simulink model "RefModel_Task"  (R2020a)
settings: Solver=ode1  StartTime=0.0  StopTime=10.0  FixedStep=Ts_Task.Ts_base  RelTol=1e-3
undefined symbols (not defined in the file or in its folder): groundspeedCmd, heightCmd, rollCmd
(part 1 of 5)
settings Model: PauseTimes=794.1  OrderedModelArguments=off  Creator=sl  LastModifiedBy=Administrator
settings DataIOCC: SaveOutput=off  SaveTime=off
settings OptimizationCC: DefaultParameterBehavior=Inlined  EnhancedBackFolding=on  PassReuseOutputArgsAs=Individual arguments  ZeroExternalMemoryAtStartup=off  ZeroInternalMemoryAtStartup=off  OptimizeBlockOrder=speed  DifferentSizesBufferReuse=on  OptimizationCustomize=off  EfficientTunableParamExpr=on
settings DebuggingCC: InheritedTsInSrcMsg=none  ParameterPrecisionLossMsg=none  ParameterTunabilityLossMsg=error  UnconnectedInputMsg=none  UnconnectedOutputMsg=none  UnconnectedLineMsg=none  SFUnusedDataAndEventsDiag=none
settings HardwareCC: ProdBitPerPointer=32  ProdBitPerSizeT=32  ProdBitPerPtrDiffT=32  ProdLargestAtomicInteger=Long  ProdLargestAtomicFloat=Double  ProdWordSize=32  ProdHWDeviceType=ARM Compatible->ARM Cortex
settings ModelReferenceCC: ModelReferenceNumInstancesAllowed=Single  PropagateVarSize=During execution
settings SFSimCC: MATLABDynamicMemAlloc=off
settings RTWCC: SystemTargetFile=ert.tlc  TemplateMakefile=ert_default_tmf  GenerateReport=on  IncludeHyperlinkInReport=on  LaunchReport=on  GenerateTraceInfo=on  GenerateTraceReport=on  GenerateTraceReportSl=on  GenerateTraceReportSf=on  GenerateTraceReportEml=on
settings CodeAppCC: ForceParamTrailComments=on  IgnoreCustomStorageClasses=off  MaxIdLength=48  OperatorAnnotations=on  SimulinkDataObjDesc=on  SFDataObjDesc=on  MATLABFcnDesc=on  InsertBlockDesc=on  StateflowObjectComments=on  MATLABSourceComments=on
settings ERTTargetCC: TargetLangStandard=C99 (ISO)  GenerateSampleERTMain=on  CombineOutputUpdateFcns=off  LogVarNameModifier=none  SupportVariableSizeSignals=on  InlinedParameterPlacement=NonHierarchical  ERTCustomFileTemplate=example_file_process.tlc

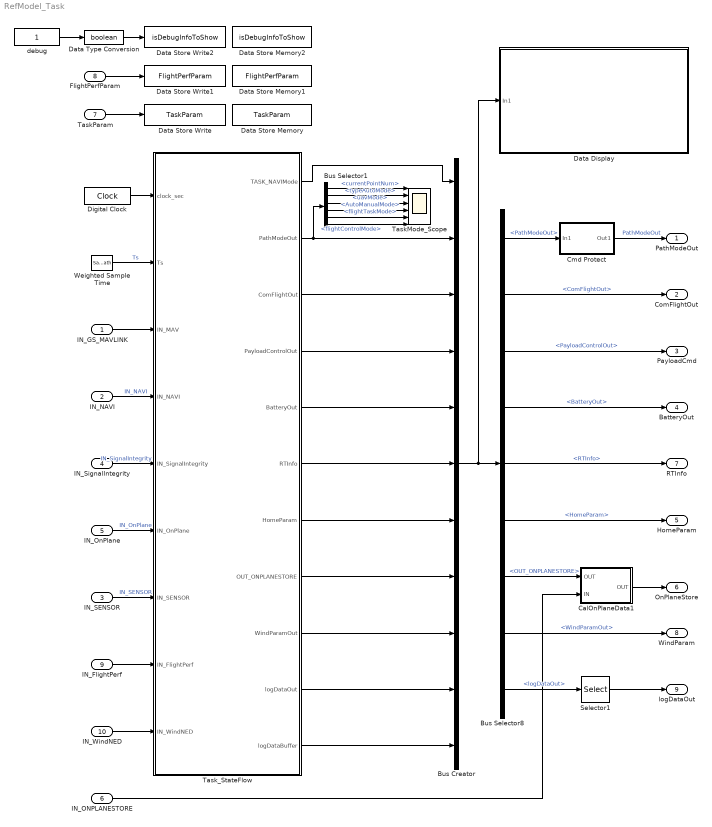
== system RefModel_Task ==
  IN_GS_MAVLINK : Inport  OutDataTypeStr=Bus: BUS_MAVLINK_TO_FIRM  BusOutputAsStruct=on
  IN_NAVI : Inport  Port=2  OutDataTypeStr=Bus: BUS_NAVI_TO_FIRM  BusOutputAsStruct=on
  IN_SENSOR : Inport  Port=3  OutDataTypeStr=Bus: BUS_SENSOR  BusOutputAsStruct=on
  IN_SignalIntegrity : Inport  Port=4  OutDataTypeStr=Bus: BUS_NAVI_SensorSignalIntegrity  BusOutputAsStruct=on
  IN_OnPlane : Inport  Port=5  OutDataTypeStr=Bus: BUS_ONPLANE_FEEDBACK  BusOutputAsStruct=on
  IN_ONPLANESTORE : Inport  Port=6  OutDataTypeStr=Bus: BUS_ONPLANE_STORE  BusOutputAsStruct=on
  TaskParam : Inport  Port=7  OutDataTypeStr=Bus: BUS_TASK_PATH_AlgoParam  BusOutputAsStruct=on
  FlightPerfParam : Inport  Port=8  OutDataTypeStr=Bus: BUS_FLIGHTPERF_PARAM  BusOutputAsStruct=on
  IN_FlightPerf : Inport  Port=9  OutDataTypeStr=Bus: BUS_FLIGHTPERF_OUT  BusOutputAsStruct=on
  IN_WindNED : Inport  Port=10  OutDataTypeStr=Bus: BUS_NAVI_GlobalWindEst
  Bus Creator : BusCreator  Inputs=11
  Bus Selector1 : BusSelector  OutputSignals=currentPointNum,typeAutoMode,uavMode,AutoManualMode,flightTaskMode,flightControlMode
  Bus Selector8 : BusSelector  OutputSignals=PathModeOut,ComFlightOut,PayloadControlOut,BatteryOut,RTInfo,HomeParam,OUT_ONPLANESTORE,WindParamOut,logDataOut
  CalOnPlaneData1 : MATLAB Function  TreatAsAtomicUnit=on
  Cmd Protect : Subsystem
  Data Display : Subsystem
      mask Display: image('$imagefile'); % Use "Edit Image" on toolstrip to change.
  Data Store Memory : DataStoreMemory  DataStoreName=TaskParam  ReadBeforeWriteMsg=warning  WriteAfterWriteMsg=warning  WriteAfterReadMsg=warning  ShowAdditionalParam=off  OutDataTypeStr=Bus: BUS_TASK_PATH_AlgoParam  Dimensions=1
  Data Store Memory1 : DataStoreMemory  DataStoreName=FlightPerfParam  ReadBeforeWriteMsg=warning  WriteAfterWriteMsg=warning  WriteAfterReadMsg=warning  ShowAdditionalParam=off  OutDataTypeStr=Bus: BUS_FLIGHTPERF_PARAM  Dimensions=1
  Data Store Memory2 : DataStoreMemory  DataStoreName=isDebugInfoToShow  ReadBeforeWriteMsg=warning  WriteAfterWriteMsg=warning  WriteAfterReadMsg=warning  ShowAdditionalParam=off  OutDataTypeStr=boolean  Dimensions=1
  Data Store Write : DataStoreWrite  DataStoreName=TaskParam
  Data Store Write1 : DataStoreWrite  DataStoreName=FlightPerfParam
  Data Store Write2 : DataStoreWrite  DataStoreName=isDebugInfoToShow
  Data Type Conversion : DataTypeConversion  OutDataTypeStr=boolean
  Digital Clock : DigitalClock  SampleTime=-1
  Selector1 : Selector  InputPortWidth=3  IndexOptions=Index vector (dialog)  Indices=1  OutputSizes=1
  TaskMode_Scope : Scope  NumInputPorts=6
  Task_StateFlow : Stateflow chart  TreatAsAtomicUnit=on
  Weighted Sample Time : SampleTimeMath  TsampMathOp=Ts Only
  debug : Constant
  PathModeOut : Outport  Description=Task模块的逻辑状态和控制指令  OutDataTypeStr=Bus: BUS_TASK_PATH_OutParam  BusOutputAsStruct=on
  ComFlightOut : Outport  Description=综合飞行参数  Port=2  OutDataTypeStr=Bus: BUS_TASK_COMMON_OutParam  BusOutputAsStruct=on
  PayloadCmd : Outport  Port=3  OutDataTypeStr=Bus: BUS_TASK_PAYLOAD  BusOutputAsStruct=on
  BatteryOut : Outport  Port=4  OutDataTypeStr=Bus: BUS_TASK_BATTERY  BusOutputAsStruct=on
  HomeParam : Outport  Port=5  OutDataTypeStr=Bus: BUS_TASK_HomeParam  BusOutputAsStruct=on
  OnPlaneStore : Outport  Port=6  OutDataTypeStr=Bus: BUS_ONPLANE_STORE  BusOutputAsStruct=on
  RTInfo : Outport  Port=7  OutDataTypeStr=Bus: BUS_TASK_RTInfo  BusOutputAsStruct=on
  " WindParam" : Outport  Port=8  OutDataTypeStr=Bus: Bus_TASK_WindParam  BusOutputAsStruct=on
  " logDataOut" : Outport  Port=9  OutDataTypeStr=Bus: BUS_TASK_SingleLog  BusOutputAsStruct=on
  wires:
  IN_GS_MAVLINK/1 -> Task_StateFlow/3(IN_MAV)
  IN_SENSOR/1 -> Task_StateFlow/7(IN_SENSOR)  "IN_SENSOR"
  IN_NAVI/1 -> Task_StateFlow/4(IN_NAVI)  "IN_NAVI"
  IN_SignalIntegrity/1 -> Task_StateFlow/5(IN_SignalIntegrity)  "IN_SignalIntegrity"
  IN_OnPlane/1 -> Task_StateFlow/6(IN_OnPlane)  "IN_OnPlane"
  Digital Clock/1 -> Task_StateFlow/1(clock_sec)
  Weighted Sample Time/1 -> Task_StateFlow/2(Ts)  "Ts"
  IN_FlightPerf/1 -> Task_StateFlow/8(IN_FlightPerf)
  IN_WindNED/1 -> Task_StateFlow/9(IN_WindNED)
  TaskParam/1 -> Data Store Write/1
  FlightPerfParam/1 -> Data Store Write1/1
  debug/1 -> Data Type Conversion/1
  Data Type Conversion/1 -> Data Store Write2/1
  Task_StateFlow/2(PathModeOut) -> Bus Selector1/1, Bus Creator/2
  Task_StateFlow/3(ComFlightOut) -> Bus Creator/3
  Task_StateFlow/4(PayloadControlOut) -> Bus Creator/4
  Task_StateFlow/5(BatteryOut) -> Bus Creator/5
  Task_StateFlow/6(RTInfo) -> Bus Creator/6
  Task_StateFlow/7(HomeParam) -> Bus Creator/7
  Task_StateFlow/8(OUT_ONPLANESTORE) -> Bus Creator/8
  Task_StateFlow/9(WindParamOut) -> Bus Creator/9
  Task_StateFlow/10(logDataOut) -> Bus Creator/10
  Task_StateFlow/11(logDataBuffer) -> Bus Creator/11
  Task_StateFlow/1(" TASK_NAVIMode") -> Bus Creator/1
  Cmd Protect/1(Out1) -> PathModeOut/1  "PathModeOut"
  CalOnPlaneData1/1(OUT) -> OnPlaneStore/1
  Bus Selector8/9 -> Selector1/1  "<logDataOut>"
  Bus Selector8/6 -> HomeParam/1  "<HomeParam>"
  Bus Selector8/3 -> PayloadCmd/1  "<PayloadControlOut>"
  Bus Selector8/7 -> CalOnPlaneData1/1("OUT ")  "<OUT_ONPLANESTORE>"
  Bus Selector8/4 -> BatteryOut/1  "<BatteryOut>"
  Bus Selector8/2 -> ComFlightOut/1  "<ComFlightOut>"
  Bus Selector8/5 -> RTInfo/1  "<RTInfo>"
  Selector1/1 -> " logDataOut"/1
  Bus Selector8/1 -> Cmd Protect/1(In1)  "<PathModeOut>"
  Bus Selector8/8 -> " WindParam"/1  "<WindParamOut>"
  Bus Creator/1 -> Data Display/1(In1), Bus Selector8/1
  IN_ONPLANESTORE/1 -> CalOnPlaneData1/2(IN)
  Bus Selector1/1 -> TaskMode_Scope/1  "<currentPointNum>"
  Bus Selector1/2 -> TaskMode_Scope/2  "<typeAutoMode>"
  Bus Selector1/3 -> TaskMode_Scope/3  "<uavMode>"
  Bus Selector1/4 -> TaskMode_Scope/4  "<AutoManualMode>"
  Bus Selector1/5 -> TaskMode_Scope/5  "<flightTaskMode>"
  Bus Selector1/6 -> TaskMode_Scope/6  "<flightControlMode>"

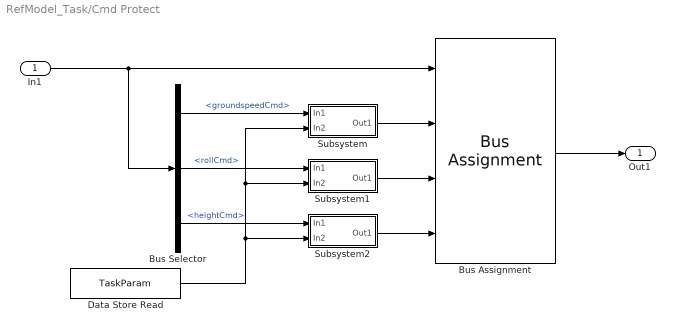
== system RefModel_Task/Cmd Protect ==
  In1 : Inport  OutDataTypeStr=Bus: BUS_TASK_PATH_OutParam
  Bus Assignment : BusAssignment  AssignedSignals=groundspeedCmd,rollCmd,heightCmd
  Bus Selector : BusSelector  OutputSignals=groundspeedCmd,rollCmd,heightCmd
  Data Store Read : DataStoreRead  DataStoreName=TaskParam
  Subsystem : Subsystem
  Subsystem1 : Subsystem
  Subsystem2 : Subsystem
  Out1 : Outport
  wires:
  In1/1 -> Bus Selector/1, Bus Assignment/1
  Bus Assignment/1 -> Out1/1
  Bus Selector/1 -> Subsystem/1(In1)  "<groundspeedCmd>"
  Bus Selector/2 -> Subsystem1/1(In1)  "<rollCmd>"
  Bus Selector/3 -> Subsystem2/1(In1)  "<heightCmd>"
  Subsystem/1(Out1) -> Bus Assignment/2
  Subsystem1/1(Out1) -> Bus Assignment/3
  Subsystem2/1(Out1) -> Bus Assignment/4
  Data Store Read/1 -> Subsystem2/2(In2), Subsystem1/2(In2), Subsystem/2(In2)

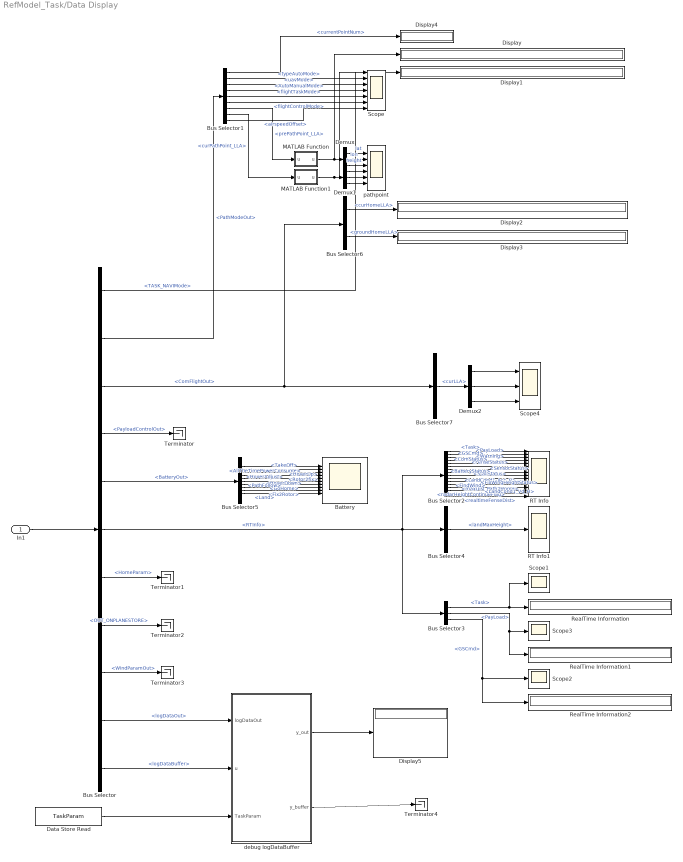
== system RefModel_Task/Data Display ==
  In1 : Inport
  Battery : Scope  NumInputPorts=10
  Bus Selector : BusSelector  OutputSignals=TASK_NAVIMode,PathModeOut,ComFlightOut,PayloadControlOut,BatteryOut,RTInfo,HomeParam,OUT_ONPLANESTORE,WindParamOut,logDataOut,logDataBuffer
  Bus Selector1 : BusSelector  OutputSignals=currentPointNum,typeAutoMode,uavMode,AutoManualMode,flightTaskMode,flightControlMode,prePathPoint_LLA,curPathPoint_LLA,airspeedOffset
  Bus Selector2 : BusSelector  OutputSignals=Task,PayLoad,GSCmd,Warning,ComStatus,FenseStatus,StallStatus,SensorStatus,BatteryStatus,FixWingHeightStatus,FindWind,LandCond1_Acc_H,LandCond1_Vd_H,radarHeightContinueFlag,maxDist_Path2Home,realtimeFenseDist
  Bus Selector3 : BusSelector  OutputSignals=Task,PayLoad,GSCmd
  Bus Selector4 : BusSelector  OutputSignals=landMaxHeight
  Bus Selector5 : BusSelector  OutputSignals=PowerConsume.AllTheTimePowerConsume,PowerConsume.TakeOff,PowerConsume.HoverAdjust,PowerConsume.Rotor2fix,PowerConsume.HoverUp,PowerConsume.PathFollow,PowerConsume.GoHome,PowerConsume.HoverDown,PowerConsume.Fix2Rotor,PowerConsume.Land
  Bus Selector6 : BusSelector  OutputSignals=curHomeLLA,groundHomeLLA
  Bus Selector7 : BusSelector  OutputSignals=curLLA
  Data Store Read : DataStoreRead  DataStoreName=TaskParam
  Demux : Demux  Outputs=3
  Demux1 : Demux  Outputs=3
  Demux2 : Demux  Outputs=3
  Display{,1..5} (6 alike) : Display
  MATLAB Function : MATLAB Function  TreatAsAtomicUnit=on
  MATLAB Function1 : MATLAB Function  TreatAsAtomicUnit=on
  RT Info : Scope  NumInputPorts=16
  RT Info1 : Scope
  RealTime Information : Display
  RealTime Information1 : Display
  RealTime Information2 : Display
  Scope : Scope  NumInputPorts=7
  Scope1 : Scope
  Scope2 : Scope
  Scope3 : Scope
  Scope4 : Scope  NumInputPorts=3
  Terminator{,1..4} (5 alike) : Terminator
  debug logDataBuffer : MATLAB Function  TreatAsAtomicUnit=on
  pathpoint : Scope  NumInputPorts=6
  wires:
  Bus Selector/2 -> Bus Selector1/1  "<PathModeOut>"
  Bus Selector3/3 -> RealTime Information2/1, Scope2/1  "<GSCmd>"
  Bus Selector5/8 -> Battery/8  "<HoverDown>"
  debug logDataBuffer/1(y_out) -> Display5/1
  Bus Selector2/2 -> RT Info/2  "<PayLoad>"
  Bus Selector4/1 -> RT Info1/1  "<landMaxHeight>"
  Bus Selector/1 -> Scope/1  "<TASK_NAVIMode>"
  Bus Selector/6 -> Bus Selector3/1, Bus Selector2/1, Bus Selector4/1  "<RTInfo>"
  Bus Selector1/5 -> Scope/5  "<flightTaskMode>"
  Bus Selector5/2 -> Battery/2  "<TakeOff>"
  Bus Selector7/1 -> Demux2/1  "<curLLA>"
  Bus Selector2/14 -> RT Info/14  "<radarHeightContinueFlag>"
  Bus Selector5/9 -> Battery/9  "<Fix2Rotor>"
  Bus Selector/3 -> Bus Selector6/1, Bus Selector7/1  "<ComFlightOut>"
  Bus Selector5/1 -> Battery/1  "<AllTheTimePowerConsume>"
  Bus Selector/10 -> debug logDataBuffer/1(logDataOut)  "<logDataOut>"
  Bus Selector/5 -> Bus Selector5/1  "<BatteryOut>"
  Bus Selector1/6 -> Scope/6  "<flightControlMode>"
  Demux2/2 -> Scope4/2
  Bus Selector2/15 -> RT Info/15  "<maxDist_Path2Home>"
  Bus Selector/11 -> debug logDataBuffer/2(u)  "<logDataBuffer>"
  Bus Selector2/6 -> RT Info/6  "<FenseStatus>"
  MATLAB Function1/1(u) -> Display1/1, Demux1/1
  Bus Selector3/2 -> RealTime Information1/1, Scope3/1  "<PayLoad>"
  Bus Selector3/1 -> RealTime Information/1, Scope1/1  "<Task>"
  Demux2/3 -> Scope4/3
  Demux/2 -> pathpoint/2  "lon"
  Bus Selector2/7 -> RT Info/7  "<StallStatus>"
  Bus Selector5/5 -> Battery/5  "<HoverUp>"
  Bus Selector2/16 -> RT Info/16  "<realtimeFenseDist>"
  Bus Selector6/1 -> Display2/1  "<curHomeLLA>"
  Bus Selector5/3 -> Battery/3  "<HoverAdjust>"
  Bus Selector5/7 -> Battery/7  "<GoHome>"
  Bus Selector5/10 -> Battery/10  "<Land>"
  Bus Selector6/2 -> Display3/1  "<groundHomeLLA>"
  Bus Selector2/4 -> RT Info/4  "<Warning>"
  Demux1/3 -> pathpoint/6
  Bus Selector5/6 -> Battery/6  "<PathFollow>"
  Bus Selector1/1 -> Display4/1  "<currentPointNum>"
  Bus Selector2/3 -> RT Info/3  "<GSCmd>"
  Bus Selector1/2 -> Scope/2  "<typeAutoMode>"
  Demux1/1 -> pathpoint/4
  Bus Selector2/12 -> RT Info/12  "<LandCond1_Acc_H>"
  Bus Selector2/1 -> RT Info/1  "<Task>"
  Bus Selector2/11 -> RT Info/11  "<FindWind>"
  Demux1/2 -> pathpoint/5
  Bus Selector5/4 -> Battery/4  "<Rotor2fix>"
  Demux2/1 -> Scope4/1
  Bus Selector2/10 -> RT Info/10  "<FixWingHeightStatus>"
  Demux/1 -> pathpoint/1  "lat"
  MATLAB Function/1(u) -> Display/1, Demux/1
  Bus Selector1/8 -> MATLAB Function1/1("u ")  "<curPathPoint_LLA>"
  Demux/3 -> pathpoint/3  "height"
  Bus Selector1/7 -> MATLAB Function/1("u ")  "<prePathPoint_LLA>"
  Bus Selector1/3 -> Scope/3  "<uavMode>"
  Bus Selector2/9 -> RT Info/9  "<BatteryStatus>"
  Bus Selector2/13 -> RT Info/13  "<LandCond1_Vd_H>"
  Bus Selector1/4 -> Scope/4  "<AutoManualMode>"
  Bus Selector2/8 -> RT Info/8  "<SensorStatus>"
  Bus Selector2/5 -> RT Info/5  "<ComStatus>"
  In1/1 -> Bus Selector/1
  debug logDataBuffer/2(y_buffer) -> Terminator4/1
  Data Store Read/1 -> debug logDataBuffer/3(TaskParam)
  Bus Selector/4 -> Terminator/1  "<PayloadControlOut>"
  Bus Selector/7 -> Terminator1/1  "<HomeParam>"
  Bus Selector/8 -> Terminator2/1  "<OUT_ONPLANESTORE>"
  Bus Selector/9 -> Terminator3/1  "<WindParamOut>"
  Bus Selector1/9 -> Scope/7  "<airspeedOffset>"

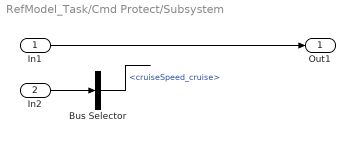
== system RefModel_Task/Cmd Protect/Subsystem ==
  In1 : Inport
  In2 : Inport  Port=2
  Bus Selector : BusSelector  OutputSignals=cruiseSpeed_cruise
  Out1 : Outport
  wires:
  In2/1 -> Bus Selector/1
  Bus Selector/1 -> ?  "<cruiseSpeed_cruise>"
  In1/1 -> Out1/1

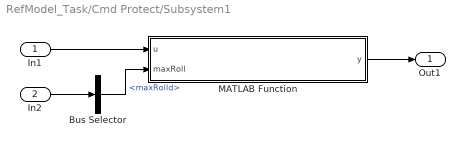
== system RefModel_Task/Cmd Protect/Subsystem1 ==
  In1 : Inport
  In2 : Inport  Port=2
  Bus Selector : BusSelector  OutputSignals=maxRolld
  MATLAB Function : MATLAB Function  TreatAsAtomicUnit=on
  Out1 : Outport
  wires:
  MATLAB Function/1(y) -> Out1/1
  Bus Selector/1 -> MATLAB Function/2(maxRoll)  "<maxRolld>"
  In2/1 -> Bus Selector/1
  In1/1 -> MATLAB Function/1(u)

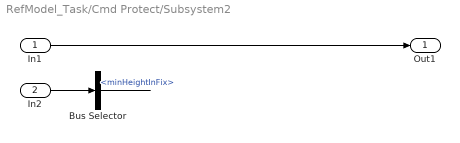
== system RefModel_Task/Cmd Protect/Subsystem2 ==
  In1 : Inport
  In2 : Inport  Port=2
  Bus Selector : BusSelector  OutputSignals=minHeightInFix
  Out1 : Outport
  wires:
  In2/1 -> Bus Selector/1
  Bus Selector/1 -> ?  "<minHeightInFix>"
  In1/1 -> Out1/1

== matlab function RefModel_Task/CalOnPlaneData1 ==
  data: OUT input Bus: BUS_ONPLANE_STORE; IN input Bus: BUS_ONPLANE_STORE; OUT output
function OUT = fcn(OUT, IN)
if IN.isDataValid
    OUT.isDataValid = IN.isDataValid;
    OUT.mileage_m = IN.mileage_m + OUT.mileage_m;
    
    OUT.Number.sortie = IN.Number.sortie + OUT.Number.sortie;
    OUT.Number.nTakeOff = IN.Number.nTakeOff + OUT.Number.nTakeOff;
    OUT.Number.nPowerOn = IN.Number.nPowerOn + OUT.Number.nPowerOn;
    OUT.Number.nPath = IN.Number.nPath + OUT.Number.nPath;
    OUT.Number.nLand = IN.Number.nLand + OUT.Number.nLand;
    OUT.Number.nRotor2Fix = IN.Number.nRotor2Fix + OUT.Number.nRotor2Fix;
    OUT.Number.nFix2Rotor = IN.Number.nFix2Rotor + OUT.Number.nFix2Rotor;
    
    OUT.Duration.fixInAir = IN.Duration.fixInAir + OUT.Duration.fixInAir;
    OUT.Duration.rotorInAir = IN.Duration.rotorInAir + OUT.Duration.rotorInAir;
    OUT.Duration.rotorOnGround = IN.Duration.rotorOnGround + OUT.Duration.rotorOnGround;
    OUT.Duration.fixAirSpeed_0_10 = IN.Duration.fixAirSpeed_0_10 + OUT.Duration.fixAirSpeed_0_10;
    OUT.Duration.fixAirSpeed_10_20 = IN.Duration.fixAirSpeed_10_20 + OUT.Duration.fixAirSpeed_10_20;
    OUT.Duration.fixAirSpeed_20_30 = IN.Duration.fixAirSpeed_20_30 + OUT.Duration.fixAirSpeed_20_30;
    OUT.Duration.fixAirSpeed_30_40 = IN.Duration.fixAirSpeed_30_40 + OUT.Duration.fixAirSpeed_30_40;
    OUT.Duration.rotorSpeed_0_5 = IN.Duration.rotorSpeed_0_5 + OUT.Duration.rotorSpeed_0_5;
    OUT.Duration.rotorSpeed_5_10 = IN.Duration.rotorSpeed_5_10 + OUT.Duration.rotorSpeed_5_10;
    OUT.Duration.rotorSpeed_10_20 = IN.Duration.rotorSpeed_10_20 + OUT.Duration.rotorSpeed_10_20;
    OUT.Duration.rotorSpeed_20_30 = IN.Duration.rotorSpeed_20_30 + OUT.Duration.rotorSpeed_20_30;
end
